simulink model "CM640C_MotAg1Meas"  (R2013b)
settings: Solver=VariableStepDiscrete  SolverMode=SingleTasking  StartTime=0.0  StopTime=1  FixedStep=0.002  RelTol=1e-3
values from neighbouring files (symbols this model uses):
  ARCHGLBPRM_2PI_ULS_F32 = DataDict.Constant    [CM640C_MotAg1Meas_DataDict.m]
  CNTPERREV_MOTREV_S15P16 = DataDict.Constant    [CM640C_MotAg1Meas_DataDict.m]
  COEFFTBLELMSIZE_CNT_U08 = DataDict.Constant    [CM640C_MotAg1Meas_DataDict.m]
  COEFFTBLSIZE_CNT_U08 = DataDict.Constant    [CM640C_MotAg1Meas_DataDict.m]
  CORRNTBLAGSTEPSIZE_MATRAD_F32 = DataDict.Constant    [CM640C_MotAg1Meas_DataDict.m]
  CORRNTBLSIDXOFFS_CNT_U16 = DataDict.Constant    [CM640C_MotAg1Meas_DataDict.m]
  CORRNTBLSIZE_CNT_U16 = DataDict.Constant    [CM640C_MotAg1Meas_DataDict.m]
  CORRNTBLSIZEMASK_CNT_U08 = DataDict.Constant    [CM640C_MotAg1Meas_DataDict.m]
  MOTAG1ERRTHD_MOTREV_U0P16 = DataDict.Constant    [CM640C_MotAg1Meas_DataDict.m]
  MotAg1MeasMotAgOffs = DataDict.Calibration    [CM640C_MotAg1Meas_DataDict.m]
  MotAg1PrtclFlt = DataDict.NTC    [CM640C_MotAg1Meas_DataDict.m]
  MOTAG1PRTCLFLTFAILSTEP_CNT_U16 = DataDict.Constant    [CM640C_MotAg1Meas_DataDict.m]
  MOTAG1PRTCLFLTPASSSTEP_CNT_U16 = DataDict.Constant    [CM640C_MotAg1Meas_DataDict.m]
  MOTAGCPTLIMFLTMASK_CNT_U32 = DataDict.Constant    [CM640C_MotAg1Meas_DataDict.m]
  MOTAGDELTAPERCORRNPT_CNT_U16 = DataDict.Constant    [CM640C_MotAg1Meas_DataDict.m]
  MOTAGFLTMASK_CNT_U32 = DataDict.Constant    [CM640C_MotAg1Meas_DataDict.m]
  MOTAGIDXMASK_CNT_U16 = DataDict.Constant    [CM640C_MotAg1Meas_DataDict.m]
  MOTAGLIMMASK_CNT_S32 = DataDict.Constant    [CM640C_MotAg1Meas_DataDict.m]
  MOTAGMGNLIMFLTMASK_CNT_U32 = DataDict.Constant    [CM640C_MotAg1Meas_DataDict.m]
  MOTAGMINWAITPERD_CNT_U32 = DataDict.Constant    [CM640C_MotAg1Meas_DataDict.m]
  MOTAGOFFS_CNT_S32 = DataDict.Constant    [CM640C_MotAg1Meas_DataDict.m]
  MOTAGOVFFLTMASK_CNT_U32 = DataDict.Constant    [CM640C_MotAg1Meas_DataDict.m]
  MOTAGSPITRSMMASK_CNT_U32 = DataDict.Constant    [CM640C_MotAg1Meas_DataDict.m]
  MOTAGVLTGFLTMASK_CNT_U32 = DataDict.Constant    [CM640C_MotAg1Meas_DataDict.m]
  NOMOTAGFLTMASK_CNT_U32 = DataDict.Constant    [CM640C_MotAg1Meas_DataDict.m]
  READBUFADR_CNT_U32 = DataDict.Constant    [CM640C_MotAg1Meas_DataDict.m]
  READBUFIDX_CNT_U08 = DataDict.Constant    [CM640C_MotAg1Meas_DataDict.m]
  SNSRAGMASK_CNT_U32 = DataDict.Constant    [CM640C_MotAg1Meas_DataDict.m]
  SNSRCNTMASK_CNT_U32 = DataDict.Constant    [CM640C_MotAg1Meas_DataDict.m]
  SPIAGCNTREGIDX_CNT_U08 = DataDict.Constant    [CM640C_MotAg1Meas_DataDict.m]
  SPIAGREGIDX_CNT_U08 = DataDict.Constant    [CM640C_MotAg1Meas_DataDict.m]
  SPISTATREGIDX_CNT_U08 = DataDict.Constant    [CM640C_MotAg1Meas_DataDict.m]
  SPITURNCNTRREGIDX_CNT_U08 = DataDict.Constant    [CM640C_MotAg1Meas_DataDict.m]
  STRTPTRINITVAL_CNT_U32 = DataDict.Constant    [CM640C_MotAg1Meas_DataDict.m]
  STRTPTRPERVAL_CNT_U32 = DataDict.Constant    [CM640C_MotAg1Meas_DataDict.m]
  TURNCNTRHALFOFFS_CNT_S16 = DataDict.Constant    [CM640C_MotAg1Meas_DataDict.m]
  TURNCNTROFFS_CNT_S16 = DataDict.Constant    [CM640C_MotAg1Meas_DataDict.m]
  TURNCNTRREGMASK_CNT_U32 = DataDict.Constant    [CM640C_MotAg1Meas_DataDict.m]
  VLDMOTAGFLTMASK_CNT_U32 = DataDict.Constant    [CM640C_MotAg1Meas_DataDict.m]
undefined symbols (not defined in the file or in its folder): NtcSts1, sigbuilder_block
libraries: simulink x41, FloatToFixd x1, NxtrMax x1
(part 6 of 7)

== system CM640C_MotAg1Meas/MotAg1Meas/MotAg1MeasPer2/MotAg1Calcn/MotAg1Processing/Diagnostics/SetParamByte/Boolean to u8  /Output 0 ==
  Action Port : ActionPort  ActionType=else
  Bit 7 : Constant  Value=0  OutDataTypeStr=uint8
  CopyRight2 : Subsystem  Description=|  mask(Copyright Information){none=on}
      | Copyright info block.                                               
      |                                                                     
      | Place copyright information at the top of every subsystem in design.
      mask prompts: none "No parameters"
      mask help: Place copyright information at the top of every subsystem in design.
      mask Display:
      | NxtrConf = 'Nexteer Confidential';
      | 
      | sys = bdroot; %handle for the current model ("system")
      | first = get_param(sys,'Created');
      | first = first(end-3:end);  %year is last four digits
      | 
      | last = get_param(sys,'LastModifiedDate');
      | if isempty(last)
      |     last = datestr(now,'yyyy');
      | else
      |     last = last(end-3:end);
      | end
      | 
      | if strcmp(first,last)
      |     fprintf('%s -- Copyright %s Nexteer',NxtrConf,first)
      | else
      |     fprintf('%s -- %s%s- %s Nexteer',NxtrConf,char(169),first,last)
      | end
  Out1 : Outport  InitialOutput=0
  wires:
  Bit 7/1 -> Out1/1

== system CM640C_MotAg1Meas/MotAg1Meas/MotAg1MeasPer2/MotAg1Calcn/MotAg1Processing/Diagnostics/SetParamByte/Boolean to u8  /Output 1 ==
  Action Port : ActionPort  ActionType=then
  Bit 7 : Constant  OutDataTypeStr=uint8
  CopyRight2 : Subsystem  Description=|  mask(Copyright Information){none=on}
      | Copyright info block.                                               
      |                                                                     
      | Place copyright information at the top of every subsystem in design.
      mask prompts: none "No parameters"
      mask help: Place copyright information at the top of every subsystem in design.
      mask Display:
      | NxtrConf = 'Nexteer Confidential';
      | 
      | sys = bdroot; %handle for the current model ("system")
      | first = get_param(sys,'Created');
      | first = first(end-3:end);  %year is last four digits
      | 
      | last = get_param(sys,'LastModifiedDate');
      | if isempty(last)
      |     last = datestr(now,'yyyy');
      | else
      |     last = last(end-3:end);
      | end
      | 
      | if strcmp(first,last)
      |     fprintf('%s -- Copyright %s Nexteer',NxtrConf,first)
      | else
      |     fprintf('%s -- %s%s- %s Nexteer',NxtrConf,char(169),first,last)
      | end
  Out1 : Outport  InitialOutput=1
  wires:
  Bit 7/1 -> Out1/1

== system CM640C_MotAg1Meas/MotAg1Meas/MotAg1MeasPer2/MotAg1Calcn/MotAg1Processing/Diagnostics/SetParamByte/Boolean to u8   /CopyRight2 ==

== system CM640C_MotAg1Meas/MotAg1Meas/MotAg1MeasPer2/MotAg1Calcn/MotAg1Processing/Diagnostics/SetParamByte/Boolean to u8   /Output 0 ==
  Action Port : ActionPort  ActionType=else
  Bit 7 : Constant  Value=0  OutDataTypeStr=uint8
  CopyRight2 : Subsystem  Description=|  mask(Copyright Information){none=on}
      | Copyright info block.                                               
      |                                                                     
      | Place copyright information at the top of every subsystem in design.
      mask prompts: none "No parameters"
      mask help: Place copyright information at the top of every subsystem in design.
      mask Display:
      | NxtrConf = 'Nexteer Confidential';
      | 
      | sys = bdroot; %handle for the current model ("system")
      | first = get_param(sys,'Created');
      | first = first(end-3:end);  %year is last four digits
      | 
      | last = get_param(sys,'LastModifiedDate');
      | if isempty(last)
      |     last = datestr(now,'yyyy');
      | else
      |     last = last(end-3:end);
      | end
      | 
      | if strcmp(first,last)
      |     fprintf('%s -- Copyright %s Nexteer',NxtrConf,first)
      | else
      |     fprintf('%s -- %s%s- %s Nexteer',NxtrConf,char(169),first,last)
      | end
  Out1 : Outport  InitialOutput=0
  wires:
  Bit 7/1 -> Out1/1

== system CM640C_MotAg1Meas/MotAg1Meas/MotAg1MeasPer2/MotAg1Calcn/MotAg1Processing/Diagnostics/SetParamByte/Boolean to u8   /Output 1 ==
  Action Port : ActionPort  ActionType=then
  Bit 7 : Constant  OutDataTypeStr=uint8
  CopyRight2 : Subsystem  Description=|  mask(Copyright Information){none=on}
      | Copyright info block.                                               
      |                                                                     
      | Place copyright information at the top of every subsystem in design.
      mask prompts: none "No parameters"
      mask help: Place copyright information at the top of every subsystem in design.
      mask Display:
      | NxtrConf = 'Nexteer Confidential';
      | 
      | sys = bdroot; %handle for the current model ("system")
      | first = get_param(sys,'Created');
      | first = first(end-3:end);  %year is last four digits
      | 
      | last = get_param(sys,'LastModifiedDate');
      | if isempty(last)
      |     last = datestr(now,'yyyy');
      | else
      |     last = last(end-3:end);
      | end
      | 
      | if strcmp(first,last)
      |     fprintf('%s -- Copyright %s Nexteer',NxtrConf,first)
      | else
      |     fprintf('%s -- %s%s- %s Nexteer',NxtrConf,char(169),first,last)
      | end
  Out1 : Outport  InitialOutput=1
  wires:
  Bit 7/1 -> Out1/1

== system CM640C_MotAg1Meas/MotAg1Meas/MotAg1MeasPer2/MotAg1Calcn/MotAg1Processing/Diagnostics/SetParamByte/Boolean to u8    /CopyRight2 ==

== system CM640C_MotAg1Meas/MotAg1Meas/MotAg1MeasPer2/MotAg1Calcn/MotAg1Processing/Diagnostics/SetParamByte/Boolean to u8    /Output 0 ==
  Action Port : ActionPort  ActionType=else
  Bit 7 : Constant  Value=0  OutDataTypeStr=uint8
  CopyRight2 : Subsystem  Description=|  mask(Copyright Information){none=on}
      | Copyright info block.                                               
      |                                                                     
      | Place copyright information at the top of every subsystem in design.
      mask prompts: none "No parameters"
      mask help: Place copyright information at the top of every subsystem in design.
      mask Display:
      | NxtrConf = 'Nexteer Confidential';
      | 
      | sys = bdroot; %handle for the current model ("system")
      | first = get_param(sys,'Created');
      | first = first(end-3:end);  %year is last four digits
      | 
      | last = get_param(sys,'LastModifiedDate');
      | if isempty(last)
      |     last = datestr(now,'yyyy');
      | else
      |     last = last(end-3:end);
      | end
      | 
      | if strcmp(first,last)
      |     fprintf('%s -- Copyright %s Nexteer',NxtrConf,first)
      | else
      |     fprintf('%s -- %s%s- %s Nexteer',NxtrConf,char(169),first,last)
      | end
  Out1 : Outport  InitialOutput=0
  wires:
  Bit 7/1 -> Out1/1

== system CM640C_MotAg1Meas/MotAg1Meas/MotAg1MeasPer2/MotAg1Calcn/MotAg1Processing/Diagnostics/SetParamByte/Boolean to u8    /Output 1 ==
  Action Port : ActionPort  ActionType=then
  Bit 7 : Constant  OutDataTypeStr=uint8
  CopyRight2 : Subsystem  Description=|  mask(Copyright Information){none=on}
      | Copyright info block.                                               
      |                                                                     
      | Place copyright information at the top of every subsystem in design.
      mask prompts: none "No parameters"
      mask help: Place copyright information at the top of every subsystem in design.
      mask Display:
      | NxtrConf = 'Nexteer Confidential';
      | 
      | sys = bdroot; %handle for the current model ("system")
      | first = get_param(sys,'Created');
      | first = first(end-3:end);  %year is last four digits
      | 
      | last = get_param(sys,'LastModifiedDate');
      | if isempty(last)
      |     last = datestr(now,'yyyy');
      | else
      |     last = last(end-3:end);
      | end
      | 
      | if strcmp(first,last)
      |     fprintf('%s -- Copyright %s Nexteer',NxtrConf,first)
      | else
      |     fprintf('%s -- %s%s- %s Nexteer',NxtrConf,char(169),first,last)
      | end
  Out1 : Outport  InitialOutput=1
  wires:
  Bit 7/1 -> Out1/1

== system CM640C_MotAg1Meas/MotAg1Meas/MotAg1MeasPer2/MotAg1Calcn/MotAg1Processing/Diagnostics/SetParamByte/Boolean to u8     /CopyRight2 ==

== system CM640C_MotAg1Meas/MotAg1Meas/MotAg1MeasPer2/MotAg1Calcn/MotAg1Processing/Diagnostics/SetParamByte/Boolean to u8     /Output 0 ==
  Action Port : ActionPort  ActionType=else
  Bit 7 : Constant  Value=0  OutDataTypeStr=uint8
  CopyRight2 : Subsystem  Description=|  mask(Copyright Information){none=on}
      | Copyright info block.                                               
      |                                                                     
      | Place copyright information at the top of every subsystem in design.
      mask prompts: none "No parameters"
      mask help: Place copyright information at the top of every subsystem in design.
      mask Display:
      | NxtrConf = 'Nexteer Confidential';
      | 
      | sys = bdroot; %handle for the current model ("system")
      | first = get_param(sys,'Created');
      | first = first(end-3:end);  %year is last four digits
      | 
      | last = get_param(sys,'LastModifiedDate');
      | if isempty(last)
      |     last = datestr(now,'yyyy');
      | else
      |     last = last(end-3:end);
      | end
      | 
      | if strcmp(first,last)
      |     fprintf('%s -- Copyright %s Nexteer',NxtrConf,first)
      | else
      |     fprintf('%s -- %s%s- %s Nexteer',NxtrConf,char(169),first,last)
      | end
  Out1 : Outport  InitialOutput=0
  wires:
  Bit 7/1 -> Out1/1

== system CM640C_MotAg1Meas/MotAg1Meas/MotAg1MeasPer2/MotAg1Calcn/MotAg1Processing/Diagnostics/SetParamByte/Boolean to u8     /Output 1 ==
  Action Port : ActionPort  ActionType=then
  Bit 7 : Constant  OutDataTypeStr=uint8
  CopyRight2 : Subsystem  Description=|  mask(Copyright Information){none=on}
      | Copyright info block.                                               
      |                                                                     
      | Place copyright information at the top of every subsystem in design.
      mask prompts: none "No parameters"
      mask help: Place copyright information at the top of every subsystem in design.
      mask Display:
      | NxtrConf = 'Nexteer Confidential';
      | 
      | sys = bdroot; %handle for the current model ("system")
      | first = get_param(sys,'Created');
      | first = first(end-3:end);  %year is last four digits
      | 
      | last = get_param(sys,'LastModifiedDate');
      | if isempty(last)
      |     last = datestr(now,'yyyy');
      | else
      |     last = last(end-3:end);
      | end
      | 
      | if strcmp(first,last)
      |     fprintf('%s -- Copyright %s Nexteer',NxtrConf,first)
      | else
      |     fprintf('%s -- %s%s- %s Nexteer',NxtrConf,char(169),first,last)
      | end
  Out1 : Outport  InitialOutput=1
  wires:
  Bit 7/1 -> Out1/1

== system CM640C_MotAg1Meas/MotAg1Meas/MotAg1MeasPer2/MotAg1Calcn/MotAg1Processing/Diagnostics/SetParamByte/Boolean to uint8/CopyRight2 ==

== system CM640C_MotAg1Meas/MotAg1Meas/MotAg1MeasPer2/MotAg1Calcn/MotAg1Processing/Diagnostics/SetParamByte/Boolean to uint8/Output 0 ==
  Action Port : ActionPort  ActionType=else
  Bit 7 : Constant  Value=0  OutDataTypeStr=uint8
  CopyRight2 : Subsystem  Description=|  mask(Copyright Information){none=on}
      | Copyright info block.                                               
      |                                                                     
      | Place copyright information at the top of every subsystem in design.
      mask prompts: none "No parameters"
      mask help: Place copyright information at the top of every subsystem in design.
      mask Display:
      | NxtrConf = 'Nexteer Confidential';
      | 
      | sys = bdroot; %handle for the current model ("system")
      | first = get_param(sys,'Created');
      | first = first(end-3:end);  %year is last four digits
      | 
      | last = get_param(sys,'LastModifiedDate');
      | if isempty(last)
      |     last = datestr(now,'yyyy');
      | else
      |     last = last(end-3:end);
      | end
      | 
      | if strcmp(first,last)
      |     fprintf('%s -- Copyright %s Nexteer',NxtrConf,first)
      | else
      |     fprintf('%s -- %s%s- %s Nexteer',NxtrConf,char(169),first,last)
      | end
  Out1 : Outport  InitialOutput=0
  wires:
  Bit 7/1 -> Out1/1

== system CM640C_MotAg1Meas/MotAg1Meas/MotAg1MeasPer2/MotAg1Calcn/MotAg1Processing/Diagnostics/SetParamByte/Boolean to uint8/Output 1 ==
  Action Port : ActionPort  ActionType=then
  Bit 7 : Constant  OutDataTypeStr=uint8
  CopyRight2 : Subsystem  Description=|  mask(Copyright Information){none=on}
      | Copyright info block.                                               
      |                                                                     
      | Place copyright information at the top of every subsystem in design.
      mask prompts: none "No parameters"
      mask help: Place copyright information at the top of every subsystem in design.
      mask Display:
      | NxtrConf = 'Nexteer Confidential';
      | 
      | sys = bdroot; %handle for the current model ("system")
      | first = get_param(sys,'Created');
      | first = first(end-3:end);  %year is last four digits
      | 
      | last = get_param(sys,'LastModifiedDate');
      | if isempty(last)
      |     last = datestr(now,'yyyy');
      | else
      |     last = last(end-3:end);
      | end
      | 
      | if strcmp(first,last)
      |     fprintf('%s -- Copyright %s Nexteer',NxtrConf,first)
      | else
      |     fprintf('%s -- %s%s- %s Nexteer',NxtrConf,char(169),first,last)
      | end
  Out1 : Outport  InitialOutput=1
  wires:
  Bit 7/1 -> Out1/1

== system CM640C_MotAg1Meas/MotAg1Meas/MotAg1MeasPer2/MotAg1Calcn/MotAg1Processing/Diagnostics/SetParamByte/Subsystem1/CopyRight2 ==

== system CM640C_MotAg1Meas/MotAg1Meas/MotAg1MeasPer2/MotAg1Calcn/MotAg1Processing/Diagnostics/SetParamByte/Subsystem1/No Fault ==
  Action Port : ActionPort  ActionType=else
  Constant : Constant  Value=0  OutDataTypeStr=uint8
  CopyRight2 : Subsystem  Description=|  mask(Copyright Information){none=on}
      | Copyright info block.                                               
      |                                                                     
      | Place copyright information at the top of every subsystem in design.
      mask prompts: none "No parameters"
      mask help: Place copyright information at the top of every subsystem in design.
      mask Display:
      | NxtrConf = 'Nexteer Confidential';
      | 
      | sys = bdroot; %handle for the current model ("system")
      | first = get_param(sys,'Created');
      | first = first(end-3:end);  %year is last four digits
      | 
      | last = get_param(sys,'LastModifiedDate');
      | if isempty(last)
      |     last = datestr(now,'yyyy');
      | else
      |     last = last(end-3:end);
      | end
      | 
      | if strcmp(first,last)
      |     fprintf('%s -- Copyright %s Nexteer',NxtrConf,first)
      | else
      |     fprintf('%s -- %s%s- %s Nexteer',NxtrConf,char(169),first,last)
      | end
  ParamByte : Outport
  wires:
  Constant/1 -> ParamByte/1

== system CM640C_MotAg1Meas/MotAg1Meas/MotAg1MeasPer2/MotAg1Calcn/MotAg1Processing/Diagnostics/SetParamByte/Subsystem1/Set ParamByte ==
  MotAg1NoAg : Inport  RequirementInfo="{'linktype_rmi_doors' '00011b54 (/ESG Group/FDD Module Requirements/EA4 Specific/CM640C_MotAg1Meas)' '#CM640C_28' 'true' 'REQ:  CM640C_28' '' } %GIDa_cb72baaa_9de1_40ef_898c_29c8f51c5596"
  MotAg1NoXY : Inport  RequirementInfo="{'linktype_rmi_doors' '00011b54 (/ESG Group/FDD Module Requirements/EA4 Specific/CM640C_MotAg1Meas)' '#CM640C_88' 'true' 'REQ:  CM640C_88' '' } %GIDa_57c4d265_80fa_43e4_b718_188b3bb05a2a"  Port=2
  MotAg1OutofLim : Inport  RequirementInfo="{'linktype_rmi_doors' '00011b54 (/ESG Group/FDD Module Requirements/EA4 Specific/CM640C_MotAg1Meas)' '#CM640C_89' 'true' 'REQ:  CM640C_89' '' } %GIDa_bfdb4256_4104_4fd1_ac80_c1b74171349b"  Port=3
  MotAg1XYOutofLim : Inport  RequirementInfo="{'linktype_rmi_doors' '00011b54 (/ESG Group/FDD Module Requirements/EA4 Specific/CM640C_MotAg1Meas)' '#CM640C_90' 'true' 'REQ:  CM640C_90' '' } %GIDa_3c4a822b_2c25_4a13_9c29_91ab92f143bb"  Port=4
  MotAg1DSPOverFlow : Inport  RequirementInfo="{'linktype_rmi_doors' '00011b54 (/ESG Group/FDD Module Requirements/EA4 Specific/CM640C_MotAg1Meas)' '#CM640C_92' 'true' 'REQ:  CM640C_92' '' } %GIDa_636d3423_941e_4142_a241_345d20101e98"  Port=5
  MotAg1VltgFlt : Inport  RequirementInfo="{'linktype_rmi_doors' '00011b54 (/ESG Group/FDD Module Requirements/EA4 Specific/CM640C_MotAg1Meas)' '#CM640C_91' 'true' 'REQ:  CM640C_91' '' } %GIDa_e14b7ac2_4b0b_4cdc_8e67_f7864e568c16"  Port=6
  MotAg1SyncErr : Inport  RequirementInfo="{'linktype_rmi_doors' '00011b54 (/ESG Group/FDD Module Requirements/EA4 Specific/CM640C_MotAg1Meas)' '#CM640C_27' 'true' 'REQ:  CM640C_27' '' } %GIDa_60fc5c8f_dddf_437e_833b_b7bb860e606f"  Port=7
  Action Port : ActionPort  ActionType=then
  Bit0 : ArithShift  RequirementInfo="{'linktype_rmi_doors' '00011b54 (/ESG Group/FDD Module Requirements/EA4 Specific/CM640C_MotAg1Meas)' '#CM640C_28' 'true' 'REQ:  CM640C_28' '' } %GIDa_d2938c81_1d7d_4033_b382_9503addd8408"
  Bit1 : ArithShift  RequirementInfo="{'linktype_rmi_doors' '00011b54 (/ESG Group/FDD Module Requirements/EA4 Specific/CM640C_MotAg1Meas)' '#CM640C_88' 'true' 'REQ:  CM640C_88' '' } %GIDa_0f96f6d6_ba0b_40ad_afb1_c7398d4fce23"  BitShiftNumber=-1
  Bit2 : ArithShift  RequirementInfo="{'linktype_rmi_doors' '00011b54 (/ESG Group/FDD Module Requirements/EA4 Specific/CM640C_MotAg1Meas)' '#CM640C_89' 'true' 'REQ:  CM640C_89' '' } %GIDa_064676c1_d292_4091_a7a2_651cd602dfdb"  BitShiftNumber=-2
  Bit3 : ArithShift  RequirementInfo="{'linktype_rmi_doors' '00011b54 (/ESG Group/FDD Module Requirements/EA4 Specific/CM640C_MotAg1Meas)' '#CM640C_90' 'true' 'REQ:  CM640C_90' '' } %GIDa_659ac5b9_ced1_4018_b074_d562764b8d3d"  BitShiftNumber=-3
  Bit4 : ArithShift  RequirementInfo="{'linktype_rmi_doors' '00011b54 (/ESG Group/FDD Module Requirements/EA4 Specific/CM640C_MotAg1Meas)' '#CM640C_92' 'true' 'REQ:  CM640C_92' '' } %GIDa_1351be20_269f_4867_9af8_6a9c9516cd75"  BitShiftNumber=-4
  Bit5 : ArithShift  RequirementInfo="{'linktype_rmi_doors' '00011b54 (/ESG Group/FDD Module Requirements/EA4 Specific/CM640C_MotAg1Meas)' '#CM640C_91' 'true' 'REQ:  CM640C_91' '' } %GIDa_4ba7e5cd_ad94_40af_a733_e26912d7282b"  BitShiftNumber=-5
  Bit6 : ArithShift  RequirementInfo="{'linktype_rmi_doors' '00011b54 (/ESG Group/FDD Module Requirements/EA4 Specific/CM640C_MotAg1Meas)' '#CM640C_27' 'true' 'REQ:  CM640C_27' '' } %GIDa_b9a77d24_8568_4827_9dbf_c443fb56efb0"  BitShiftNumber=-6
  Bitwise Operator : simulink/Logic and Bit Operations/Bitwise Operator  logicop=OR  UseBitMask=off  NumInputPorts=7  BitMask=bin2dec('11011001')  BitMaskRealWorld=Stored Integer
  CopyRight2 : Subsystem  Description=|  mask(Copyright Information){none=on}
      | Copyright info block.                                               
      |                                                                     
      | Place copyright information at the top of every subsystem in design.
      mask prompts: none "No parameters"
      mask help: Place copyright information at the top of every subsystem in design.
      mask Display:
      | NxtrConf = 'Nexteer Confidential';
      | 
      | sys = bdroot; %handle for the current model ("system")
      | first = get_param(sys,'Created');
      | first = first(end-3:end);  %year is last four digits
      | 
      | last = get_param(sys,'LastModifiedDate');
      | if isempty(last)
      |     last = datestr(now,'yyyy');
      | else
      |     last = last(end-3:end);
      | end
      | 
      | if strcmp(first,last)
      |     fprintf('%s -- Copyright %s Nexteer',NxtrConf,first)
      | else
      |     fprintf('%s -- %s%s- %s Nexteer',NxtrConf,char(169),first,last)
      | end
  ParamByte : Outport
  wires:
  MotAg1VltgFlt/1 -> Bit5/1
  MotAg1DSPOverFlow/1 -> Bit4/1
  MotAg1XYOutofLim/1 -> Bit3/1
  MotAg1OutofLim/1 -> Bit2/1
  MotAg1NoXY/1 -> Bit1/1
  MotAg1NoAg/1 -> Bit0/1
  Bit0/1 -> Bitwise Operator/1
  Bit1/1 -> Bitwise Operator/2
  Bit2/1 -> Bitwise Operator/3
  Bit3/1 -> Bitwise Operator/4
  Bitwise Operator/1 -> ParamByte/1
  Bit4/1 -> Bitwise Operator/5
  Bit5/1 -> Bitwise Operator/6
  MotAg1SyncErr/1 -> Bit6/1
  Bit6/1 -> Bitwise Operator/7

== system CM640C_MotAg1Meas/MotAg1Meas/MotAg1MeasPer2/MotAg1Calcn/MotAg1Processing/SPI  Motor Angle Calcn/Polarity Correction/Negative Polarity/CopyRight2 ==

== system CM640C_MotAg1Meas/MotAg1Meas/MotAg1MeasPer2/MotAg1Calcn/MotAg1Processing/SPI  Motor Angle Calcn/Polarity Correction/Positive Polarity/CopyRight2 ==

== system CM640C_MotAg1Meas/MotAg1Meas/MotAg1MeasPer3/Initial Check/IdleState SendTx/MotAg1Sync/Set Chip Select High/IoHwAb_SetGpioMotAg1Cs/CopyRight2 ==

== system CM640C_MotAg1Meas/MotAg1Meas/MotAg1MeasPer3/Initial Check/IdleState SendTx/MotAg1Sync/Set Chip Select Low/IoHwAb_SetGpioMotAg1Cs/CopyRight2 ==

== system CM640C_MotAg1Meas/MotAg1Meas/MotAg1MeasPer3/Initial Check/IdleState SendTx/MotAg1Sync/Wait for 2us/GetRefTmr1MicroSec32bit/CopyRight2 ==

== system CM640C_MotAg1Meas/MotAg1Meas/MotAg1MeasPer3/Initial Check/IdleState SendTx/MotAg1Sync/Wait for 2us/GetTiSpan1MicroSec32bit/CopyRight2 ==

== system CM640C_MotAg1Meas/MotAg1Meas/MotAg1MeasInit1/Compute Correction Table/NVM Ok/Calculate Correction Table/Build Wave/Reconstructed Waveform Processing/Harmonic Coefficient Processing/CopyRight2 ==

== system CM640C_MotAg1Meas/MotAg1Meas/MotAg1MeasInit1/Compute Correction Table/NVM Ok/Calculate Correction Table/Build Wave/Reconstructed Waveform Processing/Harmonic Coefficient Processing/SinCos (Use library function from NxtrMath) ==
  Theta : Inport
  1/2 : Constant  Value=0.5  OutDataTypeStr=single
  8/pi : Constant  Value=2.5464789867401123  OutDataTypeStr=single
  Add : Sum
  Add1 : Sum  Inputs=+-
  Bitwise Operator : simulink/Logic and Bit Operations/Bitwise Operator  logicop=AND  UseBitMask=on  BitMask=15  BitMaskRealWorld=Stored Integer
      settings: AttributesFormatString=|
      | BitMask:
      | %<BitMask>
  Calc Range Limited Cosine - 2 Term : Subsystem  TreatAsAtomicUnit=on
  Calc Range Limited Sine - 2 Term : Subsystem  TreatAsAtomicUnit=on
  CopyRight2 : Subsystem  Description=|  mask(Copyright Information){none=on}
      | Copyright info block.                                               
      |                                                                     
      | Place copyright information at the top of every subsystem in design.
      mask prompts: none "No parameters"
      mask help: Place copyright information at the top of every subsystem in design.
      mask Display:
      | NxtrConf = 'Nexteer Confidential';
      | 
      | sys = bdroot; %handle for the current model ("system")
      | first = get_param(sys,'Created');
      | first = first(end-3:end);  %year is last four digits
      | 
      | last = get_param(sys,'LastModifiedDate');
      | if isempty(last)
      |     last = datestr(now,'yyyy');
      | else
      |     last = last(end-3:end);
      | end
      | 
      | if strcmp(first,last)
      |     fprintf('%s -- Copyright %s Nexteer',NxtrConf,first)
      | else
      |     fprintf('%s -- %s%s- %s Nexteer',NxtrConf,char(169),first,last)
      | end
  Data Type Conversion : DataTypeConversion  OutDataTypeStr=int32
      settings: AttributesFormatString=Round Method: %<RndMeth>
  Data Type Conversion1 : DataTypeConversion  OutDataTypeStr=single
      settings: AttributesFormatString=Round Method: %<RndMeth>
  Product : Product
  Product1 : Product
  Product2 : Product
  Truth Table : Truth Table  TreatAsAtomicUnit=on
  pi/8 : Constant  Value=0.392699092626571655  OutDataTypeStr=single
  sin(22.5degrees) : Constant  Value=0.382683426141738892  OutDataTypeStr=single
  sin(45.0degrees) : Constant  Value=0.70710676908493042  OutDataTypeStr=single
  sin(67.5degrees) : Constant  Value=0.923879504203796387  OutDataTypeStr=single
  Sin : Outport
  Cos : Outport  Port=2
  wires:
  Theta/1 -> Product/1, Add1/1
  8/pi/1 -> Product/2
  Product/1 -> Add/1
  1/2/1 -> Add/2
  Add/1 -> Data Type Conversion/1
  Data Type Conversion/1 -> Data Type Conversion1/1, Bitwise Operator/1
  pi/8/1 -> Product1/1
  Data Type Conversion1/1 -> Product1/2
  Add1/1 -> Product2/2, Product2/1, Calc Range Limited Sine - 2 Term/1(Range Limited Theta)
  Product1/1 -> Add1/2
  Truth Table/1(Sin) -> Sin/1
  Bitwise Operator/1 -> Truth Table/3(ThetaIndex)
  sin(22.5degrees)/1 -> Truth Table/4(SIN225DEG_ULS_F32)
  sin(67.5degrees)/1 -> Truth Table/5(SIN675DEG_ULS_F32)
  sin(45.0degrees)/1 -> Truth Table/6(SIN450DEG_ULS_F32)
  Product2/1 -> Calc Range Limited Sine - 2 Term/2(Range Limited Theta Sqrd), Calc Range Limited Cosine - 2 Term/1(Range Limited Theta Sqrd)
  Truth Table/2(Cos) -> Cos/1
  Calc Range Limited Sine - 2 Term/1(Sin1) -> Truth Table/1(RngLimitedSin)
  Calc Range Limited Cosine - 2 Term/1(Cos1) -> Truth Table/2(RngLimitedCos)

== system CM640C_MotAg1Meas/MotAg1Meas/MotAg1MeasInit1/Compute Correction Table/NVM Ok/Calculate Correction Table/Change Correction Coordinate/Waveform Coordinate Change/Calculate Index Scale/CopyRight2 ==

== system CM640C_MotAg1Meas/MotAg1Meas/MotAg1MeasInit1/Compute Correction Table/NVM Ok/Calculate Correction Table/Change Correction Coordinate/Waveform Coordinate Change/Correction Term Found/CopyRight2 ==

== system CM640C_MotAg1Meas/MotAg1Meas/MotAg1MeasInit1/Compute Correction Table/NVM Ok/Calculate Correction Table/Change Correction Coordinate/Waveform Coordinate Change/Correction Term Not Found/CopyRight2 ==

== system CM640C_MotAg1Meas/MotAg1Meas/MotAg1MeasInit1/Compute Correction Table/NVM Ok/Calculate Correction Table/Change Correction Coordinate/Waveform Coordinate Change/Correction Term Not Found/Denominator != 0 ==
  note: (tempX - tempY) * (IndexScale - tempA) / (tempX + pitimes2 - tempA)
  note: tempY
  tempX + pitimes2 - tempA : Inport
  tempX - tempY : Inport  Port=2
  IndexScale - tempA : Inport  Port=3
  tempY : Inport  Port=4
  Action Port : ActionPort  ActionType=then
  Add4 : Sum
  CopyRight2 : Subsystem  Description=|  mask(Copyright Information){none=on}
      | Copyright info block.                                               
      |                                                                     
      | Place copyright information at the top of every subsystem in design.
      mask prompts: none "No parameters"
      mask help: Place copyright information at the top of every subsystem in design.
      mask Display:
      | NxtrConf = 'Nexteer Confidential';
      | 
      | sys = bdroot; %handle for the current model ("system")
      | first = get_param(sys,'Created');
      | first = first(end-3:end);  %year is last four digits
      | 
      | last = get_param(sys,'LastModifiedDate');
      | if isempty(last)
      |     last = datestr(now,'yyyy');
      | else
      |     last = last(end-3:end);
      | end
      | 
      | if strcmp(first,last)
      |     fprintf('%s -- Copyright %s Nexteer',NxtrConf,first)
      | else
      |     fprintf('%s -- %s%s- %s Nexteer',NxtrConf,char(169),first,last)
      | end
  "Max Table Index, Zero based1" : Bias
  Product2 : Product  Inputs=/**
  CorrTerm Not Found : Outport
  wires:
  Product2/1 -> Add4/1
  Add4/1 -> "Max Table Index, Zero based1"/1
  "Max Table Index, Zero based1"/1 -> CorrTerm Not Found/1
  tempX + pitimes2 - tempA/1 -> Product2/1
  tempX - tempY/1 -> Product2/2
  IndexScale - tempA/1 -> Product2/3
  tempY/1 -> Add4/2

== system CM640C_MotAg1Meas/MotAg1Meas/MotAg1MeasInit1/Compute Correction Table/NVM Ok/Calculate Correction Table/Change Correction Coordinate/Waveform Coordinate Change/Correction Term Not Found/Denominator == 0 ==
  Action Port : ActionPort  ActionType=else
  Constant : Constant  Value=0  OutDataTypeStr=single
  CopyRight2 : Subsystem  Description=|  mask(Copyright Information){none=on}
      | Copyright info block.                                               
      |                                                                     
      | Place copyright information at the top of every subsystem in design.
      mask prompts: none "No parameters"
      mask help: Place copyright information at the top of every subsystem in design.
      mask Display:
      | NxtrConf = 'Nexteer Confidential';
      | 
      | sys = bdroot; %handle for the current model ("system")
      | first = get_param(sys,'Created');
      | first = first(end-3:end);  %year is last four digits
      | 
      | last = get_param(sys,'LastModifiedDate');
      | if isempty(last)
      |     last = datestr(now,'yyyy');
      | else
      |     last = last(end-3:end);
      | end
      | 
      | if strcmp(first,last)
      |     fprintf('%s -- Copyright %s Nexteer',NxtrConf,first)
      | else
      |     fprintf('%s -- %s%s- %s Nexteer',NxtrConf,char(169),first,last)
      | end
  CorrTerm Not Found : Outport
  wires:
  Constant/1 -> CorrTerm Not Found/1

== system CM640C_MotAg1Meas/MotAg1Meas/MotAg1MeasInit1/Compute Correction Table/NVM Ok/Calculate Correction Table/Change Correction Coordinate/Waveform Coordinate Change/Determine Non Wrapped Correction Term/Calculate Correction Term ==
  IndexScale : Inport
  Y1 : Inport  Port=2
  Y2 : Inport  Port=3
  ReconstructedWaveform[x] : Inport  Port=4
  ReconstructedWaveform[x+1] : Inport  Port=5
  Enable : EnablePort
  Calculate Correction Term : Subsystem  TreatAsAtomicUnit=on
  CopyRight2 : Subsystem  Description=|  mask(Copyright Information){none=on}
      | Copyright info block.                                               
      |                                                                     
      | Place copyright information at the top of every subsystem in design.
      mask prompts: none "No parameters"
      mask help: Place copyright information at the top of every subsystem in design.
      mask Display:
      | NxtrConf = 'Nexteer Confidential';
      | 
      | sys = bdroot; %handle for the current model ("system")
      | first = get_param(sys,'Created');
      | first = first(end-3:end);  %year is last four digits
      | 
      | last = get_param(sys,'LastModifiedDate');
      | if isempty(last)
      |     last = datestr(now,'yyyy');
      | else
      |     last = last(end-3:end);
      | end
      | 
      | if strcmp(first,last)
      |     fprintf('%s -- Copyright %s Nexteer',NxtrConf,first)
      | else
      |     fprintf('%s -- %s%s- %s Nexteer',NxtrConf,char(169),first,last)
      | end
  Denominator == 0 : Subsystem  TreatAsAtomicUnit=on
  If : If  NumInputs=2  IfExpression=u1 == u2
  Merge : Merge
  CorrnTerm_Found : Outport
  wires:
  If/2 -> Calculate Correction Term/Action
  If/1 -> Denominator == 0/Action
  ReconstructedWaveform[x]/1 -> Calculate Correction Term/4(ReconstructedWaveform[x])
  ReconstructedWaveform[x+1]/1 -> Calculate Correction Term/5(ReconstructedWaveform[x+1])
  Y1/1 -> Calculate Correction Term/1(Y1), If/1
  Y2/1 -> If/2, Calculate Correction Term/2(Y2)
  IndexScale/1 -> Calculate Correction Term/3(IndexScale)
  Denominator == 0/1(CorrTerm Found) -> Merge/1
  Calculate Correction Term/1(CorrnTerm_Found) -> Merge/2
  Merge/1 -> CorrnTerm_Found/1

== system CM640C_MotAg1Meas/MotAg1Meas/MotAg1MeasInit1/Compute Correction Table/NVM Ok/Calculate Correction Table/Change Correction Coordinate/Waveform Coordinate Change/Determine Non Wrapped Correction Term/CopyRight2 ==

== system CM640C_MotAg1Meas/MotAg1Meas/MotAg1MeasPer2/MotAg1Calcn/MotAg1Processing/Diagnostics/ Qualifier Sts/NtcSts and DebStep Calcn/N Step/CopyRight2 ==

== system CM640C_MotAg1Meas/MotAg1Meas/MotAg1MeasPer2/MotAg1Calcn/MotAg1Processing/Diagnostics/ Qualifier Sts/NtcSts and DebStep Calcn/P Step/CopyRight2 ==

== system CM640C_MotAg1Meas/MotAg1Meas/MotAg1MeasPer2/MotAg1Calcn/MotAg1Processing/Diagnostics/Rolling Counter/Test Pass/Wrap back to 0/CopyRight2 ==

== system CM640C_MotAg1Meas/MotAg1Meas/MotAg1MeasPer2/MotAg1Calcn/MotAg1Processing/Diagnostics/Rolling Counter/Test Pass/i++/CopyRight2 ==

== system CM640C_MotAg1Meas/MotAg1Meas/MotAg1MeasPer2/MotAg1Calcn/MotAg1Processing/Diagnostics/SetParamByte/Boolean to u8/Output 0/CopyRight2 ==

== system CM640C_MotAg1Meas/MotAg1Meas/MotAg1MeasPer2/MotAg1Calcn/MotAg1Processing/Diagnostics/SetParamByte/Boolean to u8/Output 1/CopyRight2 ==

== system CM640C_MotAg1Meas/MotAg1Meas/MotAg1MeasPer2/MotAg1Calcn/MotAg1Processing/Diagnostics/SetParamByte/Boolean to u8 /Output 0/CopyRight2 ==

== system CM640C_MotAg1Meas/MotAg1Meas/MotAg1MeasPer2/MotAg1Calcn/MotAg1Processing/Diagnostics/SetParamByte/Boolean to u8 /Output 1/CopyRight2 ==

== system CM640C_MotAg1Meas/MotAg1Meas/MotAg1MeasPer2/MotAg1Calcn/MotAg1Processing/Diagnostics/SetParamByte/Boolean to u8  /Output 0/CopyRight2 ==

== system CM640C_MotAg1Meas/MotAg1Meas/MotAg1MeasPer2/MotAg1Calcn/MotAg1Processing/Diagnostics/SetParamByte/Boolean to u8  /Output 1/CopyRight2 ==

== system CM640C_MotAg1Meas/MotAg1Meas/MotAg1MeasPer2/MotAg1Calcn/MotAg1Processing/Diagnostics/SetParamByte/Boolean to u8   /Output 0/CopyRight2 ==

== system CM640C_MotAg1Meas/MotAg1Meas/MotAg1MeasPer2/MotAg1Calcn/MotAg1Processing/Diagnostics/SetParamByte/Boolean to u8   /Output 1/CopyRight2 ==

== system CM640C_MotAg1Meas/MotAg1Meas/MotAg1MeasPer2/MotAg1Calcn/MotAg1Processing/Diagnostics/SetParamByte/Boolean to u8    /Output 0/CopyRight2 ==

== system CM640C_MotAg1Meas/MotAg1Meas/MotAg1MeasPer2/MotAg1Calcn/MotAg1Processing/Diagnostics/SetParamByte/Boolean to u8    /Output 1/CopyRight2 ==

== system CM640C_MotAg1Meas/MotAg1Meas/MotAg1MeasPer2/MotAg1Calcn/MotAg1Processing/Diagnostics/SetParamByte/Boolean to u8     /Output 0/CopyRight2 ==

== system CM640C_MotAg1Meas/MotAg1Meas/MotAg1MeasPer2/MotAg1Calcn/MotAg1Processing/Diagnostics/SetParamByte/Boolean to u8     /Output 1/CopyRight2 ==

== system CM640C_MotAg1Meas/MotAg1Meas/MotAg1MeasPer2/MotAg1Calcn/MotAg1Processing/Diagnostics/SetParamByte/Boolean to uint8/Output 0/CopyRight2 ==

== system CM640C_MotAg1Meas/MotAg1Meas/MotAg1MeasPer2/MotAg1Calcn/MotAg1Processing/Diagnostics/SetParamByte/Boolean to uint8/Output 1/CopyRight2 ==

== system CM640C_MotAg1Meas/MotAg1Meas/MotAg1MeasPer2/MotAg1Calcn/MotAg1Processing/Diagnostics/SetParamByte/Subsystem1/No Fault/CopyRight2 ==

== system CM640C_MotAg1Meas/MotAg1Meas/MotAg1MeasPer2/MotAg1Calcn/MotAg1Processing/Diagnostics/SetParamByte/Subsystem1/Set ParamByte/CopyRight2 ==

== system CM640C_MotAg1Meas/MotAg1Meas/MotAg1MeasInit1/Compute Correction Table/NVM Ok/Calculate Correction Table/Build Wave/Reconstructed Waveform Processing/Harmonic Coefficient Processing/SinCos (Use library function from NxtrMath)/Calc Range Limited Cosine - 2 Term ==
  note: This block calculates the taylor series of cos to 2 terms
      |
      | Cos(x) = 1 - X^2/2!
      | Cos(x) = 1 - X^2/2
  note: X^2
  note: 1/2
  note: X^2 * (1/2)
  note: 1 - X^2 * (1/2)
  Range Limited Theta Sqrd : Inport
  CopyRight2 : Subsystem  Description=|  mask(Copyright Information){none=on}
      | Copyright info block.                                               
      |                                                                     
      | Place copyright information at the top of every subsystem in design.
      mask prompts: none "No parameters"
      mask help: Place copyright information at the top of every subsystem in design.
      mask Display:
      | NxtrConf = 'Nexteer Confidential';
      | 
      | sys = bdroot; %handle for the current model ("system")
      | first = get_param(sys,'Created');
      | first = first(end-3:end);  %year is last four digits
      | 
      | last = get_param(sys,'LastModifiedDate');
      | if isempty(last)
      |     last = datestr(now,'yyyy');
      | else
      |     last = last(end-3:end);
      | end
      | 
      | if strcmp(first,last)
      |     fprintf('%s -- Copyright %s Nexteer',NxtrConf,first)
      | else
      |     fprintf('%s -- %s%s- %s Nexteer',NxtrConf,char(169),first,last)
      | end
  One : Constant  OutDataTypeStr=single
  Product2 : Product
  Reciprocal of 2 - (1/2) : Constant  Value=0.5  OutDataTypeStr=single
  Subtract : Sum  Inputs=-+
  Cos1 : Outport
  wires:
  One/1 -> Subtract/2
  Reciprocal of 2 - (1/2)/1 -> Product2/2
  Range Limited Theta Sqrd/1 -> Product2/1
  Product2/1 -> Subtract/1
  Subtract/1 -> Cos1/1

== system CM640C_MotAg1Meas/MotAg1Meas/MotAg1MeasInit1/Compute Correction Table/NVM Ok/Calculate Correction Table/Build Wave/Reconstructed Waveform Processing/Harmonic Coefficient Processing/SinCos (Use library function from NxtrMath)/Calc Range Limited Sine - 2 Term ==
  note: Sin(x) = X * (1 - X^2 * (1/6))
  note: X
  note: 1 - X^2 * (1/6)
  note: X^2 * (1/6)
  note: 1/6
  note: X^2
  note: This block calculates the taylor series of sin to 2 terms
      |
      | Sin(x) = X - X^3/3!
      | Sin(x) = X - X^3/6
      | Sin(x) = X * (1 - X^2 * (1/6))
  Range Limited Theta : Inport
  Range Limited Theta Sqrd : Inport  Port=2
  CopyRight2 : Subsystem  Description=|  mask(Copyright Information){none=on}
      | Copyright info block.                                               
      |                                                                     
      | Place copyright information at the top of every subsystem in design.
      mask prompts: none "No parameters"
      mask help: Place copyright information at the top of every subsystem in design.
      mask Display:
      | NxtrConf = 'Nexteer Confidential';
      | 
      | sys = bdroot; %handle for the current model ("system")
      | first = get_param(sys,'Created');
      | first = first(end-3:end);  %year is last four digits
      | 
      | last = get_param(sys,'LastModifiedDate');
      | if isempty(last)
      |     last = datestr(now,'yyyy');
      | else
      |     last = last(end-3:end);
      | end
      | 
      | if strcmp(first,last)
      |     fprintf('%s -- Copyright %s Nexteer',NxtrConf,first)
      | else
      |     fprintf('%s -- %s%s- %s Nexteer',NxtrConf,char(169),first,last)
      | end
  One : Constant  OutDataTypeStr=single
  Product2 : Product
  Product4 : Product
  Reciprocal of 6 - (1/6) : Constant  Value=0.166666671633720398  OutDataTypeStr=single
  Subtract : Sum  Inputs=-+
  Sin1 : Outport
  wires:
  Product4/1 -> Sin1/1
  Subtract/1 -> Product4/2
  Product2/1 -> Subtract/1
  Range Limited Theta/1 -> Product4/1
  Range Limited Theta Sqrd/1 -> Product2/1
  Reciprocal of 6 - (1/6)/1 -> Product2/2
  One/1 -> Subtract/2

== system CM640C_MotAg1Meas/MotAg1Meas/MotAg1MeasInit1/Compute Correction Table/NVM Ok/Calculate Correction Table/Build Wave/Reconstructed Waveform Processing/Harmonic Coefficient Processing/SinCos (Use library function from NxtrMath)/CopyRight2 ==

== system CM640C_MotAg1Meas/MotAg1Meas/MotAg1MeasInit1/Compute Correction Table/NVM Ok/Calculate Correction Table/Change Correction Coordinate/Waveform Coordinate Change/Correction Term Not Found/Denominator != 0/CopyRight2 ==

== system CM640C_MotAg1Meas/MotAg1Meas/MotAg1MeasInit1/Compute Correction Table/NVM Ok/Calculate Correction Table/Change Correction Coordinate/Waveform Coordinate Change/Correction Term Not Found/Denominator == 0/CopyRight2 ==

== system CM640C_MotAg1Meas/MotAg1Meas/MotAg1MeasInit1/Compute Correction Table/NVM Ok/Calculate Correction Table/Change Correction Coordinate/Waveform Coordinate Change/Determine Non Wrapped Correction Term/Calculate Correction Term/Calculate Correction Term ==
  Y1 : Inport
  Y2 : Inport  Port=2
  IndexScale : Inport  Port=3
  ReconstructedWaveform[x] : Inport  Port=4
  ReconstructedWaveform[x+1] : Inport  Port=5
  Action Port : ActionPort  ActionType=else
  CopyRight2 : Subsystem  Description=|  mask(Copyright Information){none=on}
      | Copyright info block.                                               
      |                                                                     
      | Place copyright information at the top of every subsystem in design.
      mask prompts: none "No parameters"
      mask help: Place copyright information at the top of every subsystem in design.
      mask Display:
      | NxtrConf = 'Nexteer Confidential';
      | 
      | sys = bdroot; %handle for the current model ("system")
      | first = get_param(sys,'Created');
      | first = first(end-3:end);  %year is last four digits
      | 
      | last = get_param(sys,'LastModifiedDate');
      | if isempty(last)
      |     last = datestr(now,'yyyy');
      | else
      |     last = last(end-3:end);
      | end
      | 
      | if strcmp(first,last)
      |     fprintf('%s -- Copyright %s Nexteer',NxtrConf,first)
      | else
      |     fprintf('%s -- %s%s- %s Nexteer',NxtrConf,char(169),first,last)
      | end
  Divide : Product  Inputs=*/
  Product : Product
  Subtract : Sum  Inputs=+-
  Subtract1 : Sum  Inputs=+-
  Subtract2 : Sum  Inputs=+-
  Subtract3 : Sum
  CorrnTerm_Found : Outport
  wires:
  IndexScale/1 -> Subtract1/1
  Y2/1 -> Subtract/1
  Y1/1 -> Subtract1/2, Subtract/2
  Subtract1/1 -> Divide/1
  Subtract/1 -> Divide/2
  Divide/1 -> Product/1
  ReconstructedWaveform[x+1]/1 -> Subtract2/1
  ReconstructedWaveform[x]/1 -> Subtract2/2, Subtract3/2
  Subtract2/1 -> Product/2
  Product/1 -> Subtract3/1
  Subtract3/1 -> CorrnTerm_Found/1

== system CM640C_MotAg1Meas/MotAg1Meas/MotAg1MeasInit1/Compute Correction Table/NVM Ok/Calculate Correction Table/Change Correction Coordinate/Waveform Coordinate Change/Determine Non Wrapped Correction Term/Calculate Correction Term/CopyRight2 ==

== system CM640C_MotAg1Meas/MotAg1Meas/MotAg1MeasInit1/Compute Correction Table/NVM Ok/Calculate Correction Table/Change Correction Coordinate/Waveform Coordinate Change/Determine Non Wrapped Correction Term/Calculate Correction Term/Denominator == 0 ==
  Action Port : ActionPort  ActionType=then
  Constant : Constant  Value=0  OutDataTypeStr=single
  CopyRight2 : Subsystem  Description=|  mask(Copyright Information){none=on}
      | Copyright info block.                                               
      |                                                                     
      | Place copyright information at the top of every subsystem in design.
      mask prompts: none "No parameters"
      mask help: Place copyright information at the top of every subsystem in design.
      mask Display:
      | NxtrConf = 'Nexteer Confidential';
      | 
      | sys = bdroot; %handle for the current model ("system")
      | first = get_param(sys,'Created');
      | first = first(end-3:end);  %year is last four digits
      | 
      | last = get_param(sys,'LastModifiedDate');
      | if isempty(last)
      |     last = datestr(now,'yyyy');
      | else
      |     last = last(end-3:end);
      | end
      | 
      | if strcmp(first,last)
      |     fprintf('%s -- Copyright %s Nexteer',NxtrConf,first)
      | else
      |     fprintf('%s -- %s%s- %s Nexteer',NxtrConf,char(169),first,last)
      | end
  CorrTerm Found : Outport
  wires:
  Constant/1 -> CorrTerm Found/1

== system CM640C_MotAg1Meas/MotAg1Meas/MotAg1MeasInit1/Compute Correction Table/NVM Ok/Calculate Correction Table/Build Wave/Reconstructed Waveform Processing/Harmonic Coefficient Processing/SinCos (Use library function from NxtrMath)/Calc Range Limited Cosine - 2 Term/CopyRight2 ==

== system CM640C_MotAg1Meas/MotAg1Meas/MotAg1MeasInit1/Compute Correction Table/NVM Ok/Calculate Correction Table/Build Wave/Reconstructed Waveform Processing/Harmonic Coefficient Processing/SinCos (Use library function from NxtrMath)/Calc Range Limited Sine - 2 Term/CopyRight2 ==

== system CM640C_MotAg1Meas/MotAg1Meas/MotAg1MeasInit1/Compute Correction Table/NVM Ok/Calculate Correction Table/Change Correction Coordinate/Waveform Coordinate Change/Determine Non Wrapped Correction Term/Calculate Correction Term/Calculate Correction Term/CopyRight2 ==

== system CM640C_MotAg1Meas/MotAg1Meas/MotAg1MeasInit1/Compute Correction Table/NVM Ok/Calculate Correction Table/Change Correction Coordinate/Waveform Coordinate Change/Determine Non Wrapped Correction Term/Calculate Correction Term/Denominator == 0/CopyRight2 ==

== stateflow chart CM640C_MotAg1Meas/MotAg1Meas/MotAg1MeasPer1/Motor Angle Processing/Offset /Chart ==
  (default) -> (junction 8) : {
      | MechMtrPos1_Out = MechMtrPos1_In;
      | }
  (junction 12) -> (junction 8)
  (junction 3) -> (junction 8)
  (junction 8) -> (junction 12) [order 1] : [
      | MechMtrPos1_Out < 0
      | ]
      | {
      | MechMtrPos1_Out = MechMtrPos1_Out + 65536;
      | }
  (junction 8) -> (junction 3) [order 2] : [
      | MechMtrPos1_Out > 65535
      | ]
      | {
      | MechMtrPos1_Out = MechMtrPos1_Out - 65536;
      | }
  (junction 8) -> (junction 1) [order 3]
  data: MechMtrPos1_In input int32; MechMtrPos1_Out output int32

== stateflow chart CM640C_MotAg1Meas/MotAg1Meas/MotAg1MeasPer1/Motor Angle Processing/Offset /Compensate MechMotPos/Chart ==
  (default) -> (junction 8) : {
      | MechMtrPos1_Out = MechMtrPos1_In;
      | }
  (junction 12) -> (junction 8)
  (junction 3) -> (junction 8)
  (junction 8) -> (junction 12) [order 1] : [
      | MechMtrPos1_Out < 0
      | ]
      | {
      | MechMtrPos1_Out = MechMtrPos1_Out + 65536;
      | }
  (junction 8) -> (junction 3) [order 2] : [
      | MechMtrPos1_Out > 65535
      | ]
      | {
      | MechMtrPos1_Out = MechMtrPos1_Out - 65536;
      | }
  (junction 8) -> (junction 1) [order 3]
  data: MechMtrPos1_In input int32; MechMtrPos1_Out output int32
